simulink model "tp405098"  (Simulink 3.0)
settings: Solver=ode1  StartTime=0.0  StopTime=time(end)  FixedStep=Ts  RelTol=1e-3
values from neighbouring files (symbols this model uses):
  Ks = input('Put integrator gain value Ks = ')    [init_PI1_windupless.m]    (also in init_PID1_windupless_tune3.m)
  T1 = input('Put time constant T1 value = ')    [init_PID1_windupless_tune3.m]
  T2 = 1    [init_PID1_windupless_tune3.m]
  Td = input('Put identified transport delay value Td = ')    [init_PI1_windupless.m]    (also in init_PID1_windupless_tune3.m = input('Put identified transport delay Td = '))
  Tfd = input('feasibility and filtration (T1/5) = ')    [init_PID1_windupless_tune3.m]
  u0 = mean(u(t_prep_in-10:t_prep_in,2))    [init_step_resp2.m]
  u_step = 4    [init_step_resp2.m]
undefined symbols (not defined in the file or in its folder): a, inp
settings Model: LastModifiedBy=mato  ExtModeTrigMode=oneshot  ExtModeArmWhenConnect=off  SaveFormat=Matrix

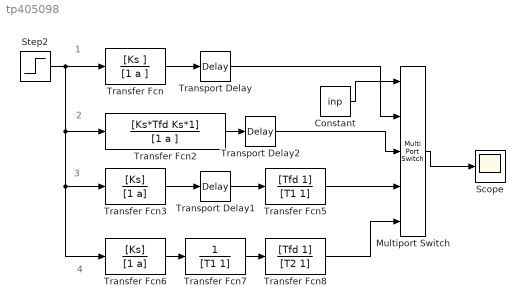
== system tp405098 ==
  note: 1
  note: 2
  note: 3
  note: 4
  Constant : Constant  Value=inp
  Multiport Switch : MultiPortSwitch  Inputs=4
  Scope : Scope
      settings: TimeRange=auto  YMin=-5  YMax=5  SaveName=y_sim  DataFormat=Matrix
  Step2 : Step  Time=0  Before=0  After=u_step-u0  SampleTime=0
  Transfer Fcn : TransferFcn  Numerator=[Ks ]  Denominator=[1 a ]
  Transfer Fcn2 : TransferFcn  Numerator=[Ks*Tfd Ks*1]  Denominator=[1 a ]
  Transfer Fcn3 : TransferFcn  Numerator=[Ks]  Denominator=[1 a]
  Transfer Fcn5 : TransferFcn  Numerator=[Tfd 1]  Denominator=[T1 1]
  Transfer Fcn6 : TransferFcn  Numerator=[Ks]  Denominator=[1 a]
  Transfer Fcn7 : TransferFcn  Numerator=1  Denominator=[T1 1]
  Transfer Fcn8 : TransferFcn  Numerator=[Tfd 1]  Denominator=[T2 1]
  Transport Delay : TransportDelay  DelayTime=Td  InitialInput=0  BufferSize=1024
  Transport Delay1 : TransportDelay  DelayTime=Td  InitialInput=0  BufferSize=1024
  Transport Delay2 : TransportDelay  DelayTime=Td  InitialInput=0  BufferSize=1024
  wires:
  Transfer Fcn/1 -> Transport Delay/1
  Step2/1 -> Transfer Fcn/1, Transfer Fcn3/1, Transfer Fcn6/1, Transfer Fcn2/1
  Transfer Fcn2/1 -> Transport Delay2/1
  Transport Delay/1 -> Multiport Switch/2
  Transfer Fcn3/1 -> Transport Delay1/1
  Transport Delay1/1 -> Transfer Fcn5/1
  Constant/1 -> Multiport Switch/1
  Transport Delay2/1 -> Multiport Switch/3
  Transfer Fcn5/1 -> Multiport Switch/4
  Multiport Switch/1 -> Scope/1
  Transfer Fcn6/1 -> Transfer Fcn7/1
  Transfer Fcn7/1 -> Transfer Fcn8/1
  Transfer Fcn8/1 -> Multiport Switch/5
